simulink model "simulinkcsvkibam"  (R2018b)
settings: Solver=VariableStepAuto  StartTime=0.0  StopTime=86400  RelTol=1e-3
model workspace (MAT data in the model file):
  c = 0.5
  capacity = 119808000
  p = 0.1
  ub = 149760000
libraries: simulink x1
settings Model: Creator=mathis  LastModifiedBy=Hvati
settings DebuggingCC: LibraryContextMissingDiagnostic=none
settings SFSimCC: SimUseLocalCustomCode=off
settings RTWCC: RTWUseLocalCustomCode=off

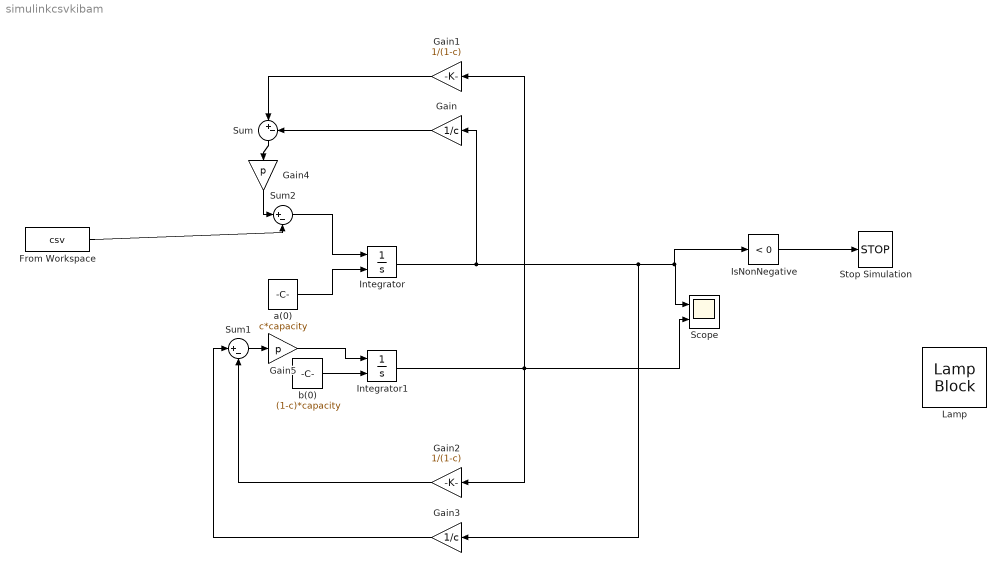
== system simulinkcsvkibam ==
  From Workspace : FromWorkspace  VariableName=csv  SampleTime=0
  Gain : Gain  Gain=1/c
  Gain1 : Gain  Gain=1/(1-c)
  Gain2 : Gain  Gain=1/(1-c)
  Gain3 : Gain  Gain=1/c
  Gain4 : Gain  Gain=p
  Gain5 : Gain  Gain=p
  Integrator : Integrator  InitialConditionSource=external  LimitOutput=on  UpperSaturationLimit=c*149760000
  Integrator1 : Integrator  InitialConditionSource=external
  IsNonNegative : simulink/Logic and Bit Operations/Compare To Zero  relop=<  OutDataTypeStr=boolean  ZeroCross=off
  Lamp : LampBlock  WebBlockId=25
  Scope : Scope  NumInputPorts=2
  Stop Simulation : Stop
  Sum : Sum  Inputs=|+-
  Sum1 : Sum  Inputs=|+-
  Sum2 : Sum  Inputs=|+-
  a(0) : Constant  Value=c*capacity
  b(0) : Constant  Value=(1-c)*capacity
  wires:
  b(0)/1 -> Integrator1/2
  a(0)/1 -> Integrator/2
  Gain/1 -> Sum/2
  Integrator/1 -> Gain3/1, IsNonNegative/1, Scope/1, Gain/1
  Gain1/1 -> Sum/1
  Integrator1/1 -> Scope/2, Gain2/1, Gain1/1
  Sum/1 -> Gain4/1
  Sum1/1 -> Gain5/1
  Gain2/1 -> Sum1/2
  Gain3/1 -> Sum1/1
  Sum2/1 -> Integrator/1
  Gain4/1 -> Sum2/1
  Gain5/1 -> Integrator1/1
  IsNonNegative/1 -> Stop Simulation/1
  From Workspace/1 -> Sum2/2
